simulink model "Proj_5_part_1"  (R2016b)
settings: Solver=ode4  StartTime=0.0  StopTime=200  FixedStep=0.01  RelTol=1e-3
settings Model: Creator=apple  LastModifiedBy=apple

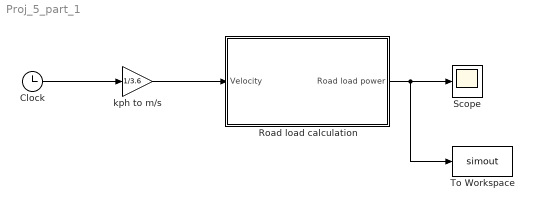
== system Proj_5_part_1 ==
  Clock : Clock
  Road load calculation : Subsystem
  Scope : Scope
  To Workspace : ToWorkspace  VariableName=simout  SaveFormat=Timeseries  SampleTime=-1
  kph to m/s : Gain  Gain=1/3.6
  wires:
  Clock/1 -> kph to m/s/1
  kph to m/s/1 -> Road load calculation/1(Velocity)
  Road load calculation/1(Road load power) -> To Workspace/1, Scope/1

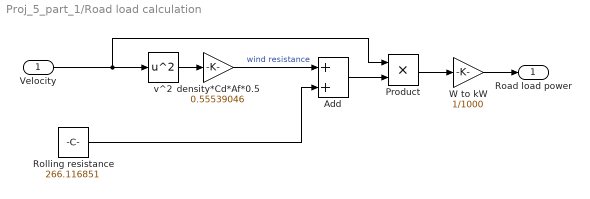
== system Proj_5_part_1/Road load calculation ==
  Velocity : Inport
  Add : Sum
  Product : Product
  Rolling resistance : Constant  Value=266.116851
  W to kW : Gain  Gain=1/1000
  density*Cd*Af*0.5 : Gain  Gain=0.55539046
  v^2 : Math  Operator=square  SaturateOnIntegerOverflow=on
  Road load power : Outport
  wires:
  Product/1 -> W to kW/1
  W to kW/1 -> Road load power/1
  Velocity/1 -> Product/1, v^2/1
  density*Cd*Af*0.5/1 -> Add/1  "wind resistance"
  v^2/1 -> density*Cd*Af*0.5/1
  Rolling resistance/1 -> Add/2
  Add/1 -> Product/2
